simulink model "Backstepping_DELTA"  (R2018b)
settings: Solver=FixedStepAuto  StartTime=0.0  StopTime=25  FixedStep=0.0001  RelTol=1e-5
model workspace (MAT data in the model file):
  I_bc = 0.466666666667
  I_bi = 2.46666666667
  I_brake = 1
  I_m = 1
  R = 0.63
  b = 2
  ee = [0; 0; -2.1944]
  k_r = 1
  l_A = 1
  l_B = 2
  m_b = 1
  m_br = 1.13333333333
  m_c = 0
  m_fb = 0.2
  m_n = 1
  m_nt = 3.6
  m_p = 0
  r_Gb = 0.558823529412
  r_l = 0.63
  r_m = 0.666666666667
  theta = [0 2.09439510239 4.18879020479]
settings Model: Creator=enrico  LastModifiedBy=Dan

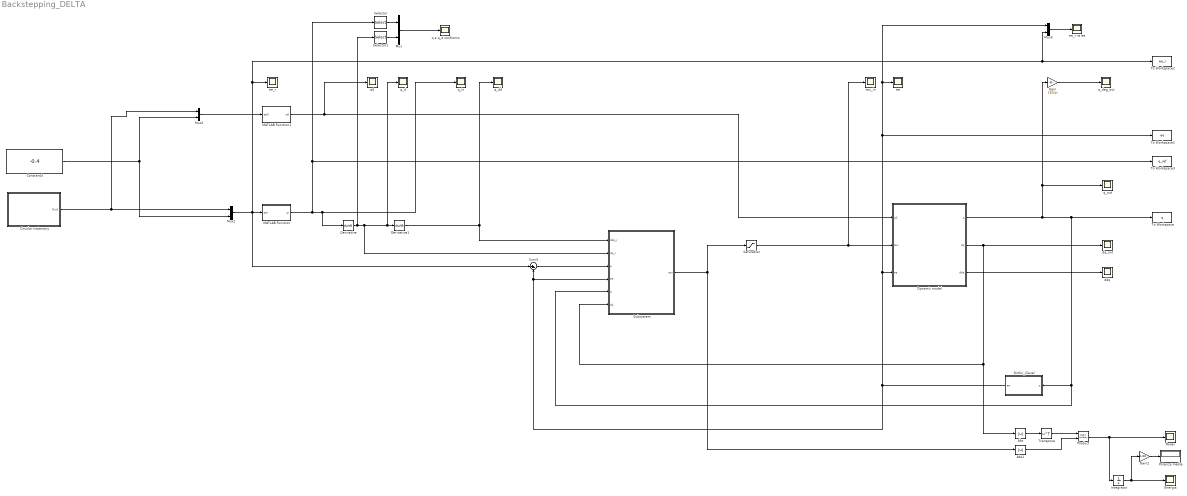
== system Backstepping_DELTA ==
  Abs : Abs
  Abs1 : Abs
  Circular trajectory : Subsystem  mask{A=0.05, F=3}
      mask prompts: A "Amplitude"; F "Frequency"
  Constant3 : Constant  Value=-0.4  SampleTime=-1
  Derivative : Derivative
  Derivative1 : Derivative
  DirKin_Clavel : MATLAB Function  TreatAsAtomicUnit=on
      mask init:
      | loadvar
  Dynamic model : Subsystem
  Energia : Scope
  Gain : Gain  Gain=180/pi
  Gain2 : Gain  Gain=1/10
  Integrator : Integrator
  MATLAB Function : MATLAB Function  TreatAsAtomicUnit=on
  MATLAB Function1 : MATLAB Function  TreatAsAtomicUnit=on
  Mux{,1..3} (4 alike) : Mux  Inputs=2
  Potenza media : Display
  Power : Scope
  Product : Product  Multiplication=Matrix(*)
  Saturation : Saturate  UpperLimit=20  LowerLimit=-20  ZeroCross=off
  Selector : Selector  InputPortWidth=3  IndexOptions=Index vector (dialog)  Indices=[1]  OutputSizes=1
  Selector1 : Selector  InputPortWidth=3  IndexOptions=Index vector (dialog)  Indices=[1]  OutputSizes=1
  Subsystem : Subsystem  mask{K_l=400, K_d=50}
      mask prompts: K_l "Kinematic control gain"; K_d "Derivative_gain"
  Sum3 : Sum  Inputs=|+-
  To Workspace : ToWorkspace  VariableName=q  SampleTime=-1
  To Workspace1 : ToWorkspace  VariableName=ee  SampleTime=-1
  To Workspace2 : ToWorkspace  VariableName=ee_r  SampleTime=-1
  To Workspace3 : ToWorkspace  VariableName=q_ref  SampleTime=-1
  Transpose : Math  Operator=transpose  SaturateOnIntegerOverflow=on
  ddq : Scope
  "dq_out " : Scope
  "ee " : Scope
  ee_r : Scope
  ee_r vs ee : Scope
  q e q_d confronto : Scope
  "q0 " : Scope
  "q_d " : Scope
  q_dd : Scope
  "q_deg_out " : Scope
  q_in : Scope
  q_out : Scope
  tau_in : Scope
  wires:
  Gain/1 -> "q_deg_out "/1
  Dynamic model/3(ddq) -> ddq/1
  Dynamic model/1(q) -> q_out/1, Gain/1, Subsystem/5(q), DirKin_Clavel/1(q), To Workspace/1
  MATLAB Function1/1(q0) -> Dynamic model/1("q0 "), "q0 "/1
  Mux2/1 -> MATLAB Function1/1(ee0)
  Constant3/1 -> Mux1/2, Mux2/2
  Dynamic model/2(dq) -> Abs/1, Subsystem/6(dq), "dq_out "/1
  Subsystem/1(tau) -> Saturation/1, Abs1/1
  Derivative1/1 -> q_dd/1, Subsystem/1(ddq_r)
  Product/1 -> Integrator/1, Power/1
  Transpose/1 -> Product/1
  Abs/1 -> Transpose/1
  Abs1/1 -> Product/2
  Mux/1 -> q e q_d confronto/1
  Selector/1 -> Mux/1
  Selector1/1 -> Mux/2
  MATLAB Function/1(qr) -> Selector/1, To Workspace3/1, q_in/1, Derivative/1
  Derivative/1 -> Derivative1/1, "q_d "/1, Subsystem/2(dq_r), Selector1/1
  DirKin_Clavel/1(ee) -> Mux3/1, "ee "/1, To Workspace1/1, Dynamic model/3(ee), Sum3/2, Subsystem/4(ee)
  Mux3/1 -> ee_r vs ee/1
  Mux1/1 -> MATLAB Function/1(eer), Sum3/1, ee_r/1, To Workspace2/1, Mux3/2
  Integrator/1 -> Gain2/1, Energia/1
  Circular trajectory/1(Out1) -> Mux1/1, Mux2/1
  Gain2/1 -> Potenza media/1
  Sum3/1 -> Subsystem/3(e)
  Saturation/1 -> tau_in/1, Dynamic model/2(tau)

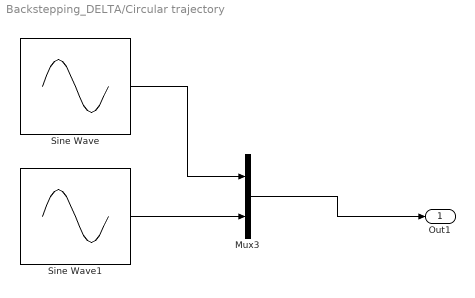
== system Backstepping_DELTA/Circular trajectory ==
  Mux3 : Mux  Inputs=2
  Sine Wave : Sin  Amplitude=A  Frequency=F  Phase=pi/2
  Sine Wave1 : Sin  Amplitude=A  Frequency=F
  Out1 : Outport
  wires:
  Mux3/1 -> Out1/1
  Sine Wave/1 -> Mux3/1
  Sine Wave1/1 -> Mux3/2

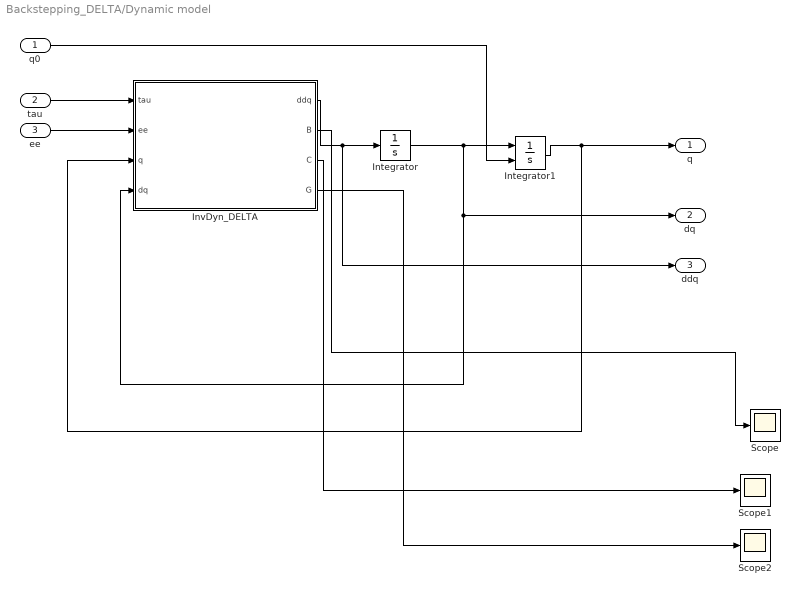
== system Backstepping_DELTA/Dynamic model ==
  "q0 " : Inport
  tau : Inport  Port=2
  ee : Inport  Port=3
  Integrator : Integrator  InitialCondition=[0; 0; 0]
  Integrator1 : Integrator  InitialConditionSource=external  InitialCondition=[pi/4; pi/4; pi/4]
  InvDyn_DELTA : MATLAB Function  TreatAsAtomicUnit=on
  Scope : Scope
  Scope1 : Scope
  Scope2 : Scope
  q : Outport
  dq : Outport  Port=2
  ddq : Outport  Port=3
  wires:
  InvDyn_DELTA/1(ddq) -> ddq/1, Integrator/1
  ee/1 -> InvDyn_DELTA/2(ee)
  Integrator1/1 -> q/1, InvDyn_DELTA/3(q)
  Integrator/1 -> Integrator1/1, dq/1, InvDyn_DELTA/4(dq)
  tau/1 -> InvDyn_DELTA/1(tau)
  "q0 "/1 -> Integrator1/2
  InvDyn_DELTA/2(B) -> Scope/1
  InvDyn_DELTA/3(C) -> Scope1/1
  InvDyn_DELTA/4(G) -> Scope2/1

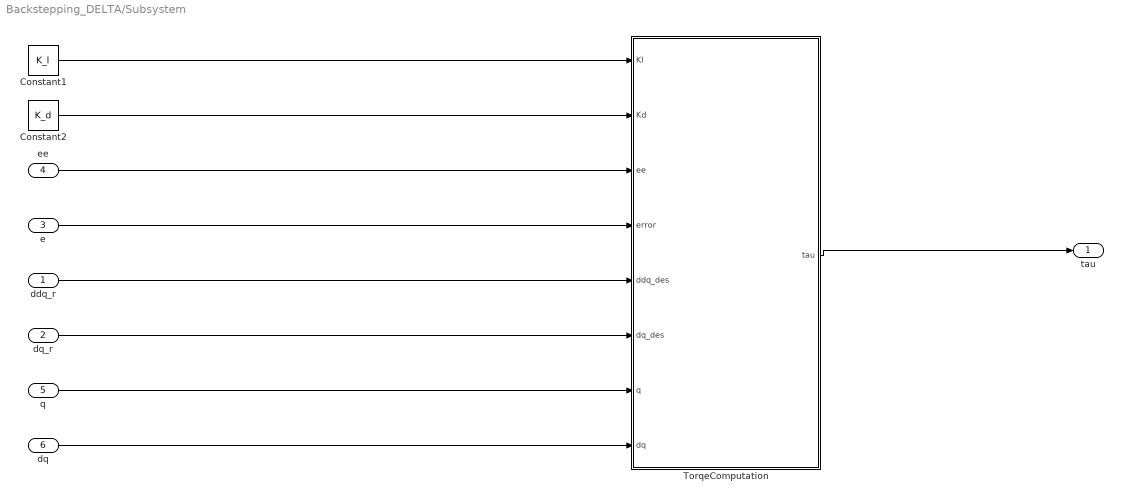
== system Backstepping_DELTA/Subsystem ==
  ddq_r : Inport
  dq_r : Inport  Port=2
  e : Inport  Port=3
  ee : Inport  Port=4
  q : Inport  Port=5
  dq : Inport  Port=6
  Constant1 : Constant  Value=K_l
  Constant2 : Constant  Value=K_d
  TorqeComputation : MATLAB Function  TreatAsAtomicUnit=on
  tau : Outport
  wires:
  ddq_r/1 -> TorqeComputation/5(ddq_des)
  e/1 -> TorqeComputation/4(error)
  q/1 -> TorqeComputation/7(q)
  TorqeComputation/1(tau) -> tau/1
  ee/1 -> TorqeComputation/3(ee)
  dq_r/1 -> TorqeComputation/6(dq_des)
  dq/1 -> TorqeComputation/8(dq)
  Constant1/1 -> TorqeComputation/1(Kl)
  Constant2/1 -> TorqeComputation/2(Kd)

== matlab function Backstepping_DELTA/MATLAB Function1 ==
  data: ee0 input; q0 output
function q0 = InverseKinematic(ee0)
%Computation of the inverse kinematic of the Delta robot

% Loading parameters
[theta, R, ~, ~, l_A, ~, ~, l_B, ~, ~, ~] = Parameters_DELTA;

R_b1 = R_base(theta(1));
R_b2 = R_base(theta(2));
R_b3 = R_base(theta(3));
p = [R_b1\ee0, R_b2\ee0, R_b3\ee0]; 
q0 = nan(3,1);

for li=1:3
    
    x0 = p(1,li);
    y0 = p(2,li);
    z0 = p(3,li);
    A = l_A^2 - l_B^2 - R^2 + x0^2 + y0^2 + z0^2;
    B = 2*x0 - 2*R;

    a = 4*z0^2 + B^2;
    b = 4*R*z0^2 + A*B;
    c = A^2 + 4*R^2*z0^2 - 4*l_A^2*z0^2;
        
    x = (b + sqrt(b^2 - a*c))/a; 
    
    z = (A - B*x)/(2*z0);
    
    q0(li) = - asin(z/l_A); 
    
    if x-R < 0
        q0(li) = pi - q0(li);
    end    
end

end

== matlab function Backstepping_DELTA/Dynamic model/InvDyn_DELTA ==
  data: tau input; ddq output; ee input; q input; dq input; B output; C output; G output
function [ddq, B, C, G] = InvDyn_DELTA(tau, ee, q, dq)
% References:
% [1] Olsson, A. (2009). Modelling and control of a Delta-3 robot, (February).
% [2] Codourey, A. (1998). Dynamic Modeling of Parallel Robots for Computed-Torque Control Implementation, 17(12), 1325–1336.

% B, C, G matrices
[B, C, G, F] = BCG_DELTA(ee,q);


% Inverse dynamic
ddq = B\(tau - C*dq - G - F*dq); % Think adding friction coefficient of the manipulator (from [1] pg 27) 


end

== matlab function Backstepping_DELTA/DirKin_Clavel ==
  data: q input; ee output
function ee = DirKin_Clavel(q)

[theta, R, ~, ~, l_A, ~, ~, l_B, ~, ~, ~] = Parameters_DELTA;

D = nan(3,1);
E = nan(3,1);
F = nan(3,1);
G = nan(3,1);

for i = 1:3
   D(i) = -l_B^2 + l_A^2 + R^2 + 2*R*l_A*cos(q(i));
   
   E(i) = 2*(R + l_A*cos(q(i)))*cos(theta(i));
   
   F(i) = 2*(R + l_A*cos(q(i)))*sin(theta(i));
   
   G(i) = -2*l_A*sin(q(i)); 
end

H = [E(1)*G(2) - E(1)*G(3) - E(2)*G(1) + E(2)*G(3) + E(3)*G(1) - E(3)*G(2);
    -E(1)*F(2) + E(1)*F(3) + E(2)*F(1) - E(2)*F(3) - E(3)*F(1) + E(3)*F(2);
    -E(1)*D(2) + E(1)*D(3) + E(2)*D(1) - E(2)*D(3) - E(3)*D(1) + E(3)*D(2);
     F(1)*D(2) - F(1)*D(3) - F(2)*D(1) + F(2)*D(3) + F(3)*D(1) - F(3)*D(2);
    -F(1)*G(2) + F(1)*G(3) + F(2)*G(1) - F(2)*G(3) - F(3)*G(1) + F(3)*G(2)];

L = (H(5)^2 + H(1)^2)/H(2)^2 + 1;

M = 2*(H(5)*H(4) + H(1)*H(3))/H(2)^2 - (H(5)*E(1) + H(1)*F(1))/H(2) - G(1);

N = (H(4)^2 + H(3)^2)/H(2)^2 - (H(4)*E(1) + H(3)*F(1))/H(2) + D(1);

ee = nan(3,1);
ee2 = nan(3,1);

ee(3) = (-M + sqrt(M^2 - 4*L*N))/(2*L);

ee(1) = ee(3)*H(5)/H(2) + H(4)/H(2);

ee(2) = ee(3)*H(1)/H(2) + H(3)/H(2);

ee2(3) = (-M - sqrt(M^2 - 4*L*N))/(2*L);

ee2(1) = ee2(3)*H(5)/H(2) + H(4)/H(2);

ee2(2) = ee2(3)*H(1)/H(2) + H(3)/H(2);
 


% if ee2(3) < 0 
%     ee = ee2;
% end

if ee(3) > ee2(3)
    ee = ee2;
end

end

== matlab function Backstepping_DELTA/MATLAB Function ==
  data: eer input; qr output
function qr = InverseKinematic(eer)
%Computation of the inverse kinematic of the Delta robot

% Loading parameters
[theta, R, ~, ~, l_A, ~, ~, l_B, ~, ~, ~] = Parameters_DELTA;

R_b1 = R_base(theta(1));
R_b2 = R_base(theta(2));
R_b3 = R_base(theta(3));
p = [R_b1\eer, R_b2\eer, R_b3\eer]; 
qr = nan(3,1);

for li=1:3
    
    x0 = p(1,li);
    y0 = p(2,li);
    z0 = p(3,li);
    A = l_A^2 - l_B^2 - R^2 + x0^2 + y0^2 + z0^2;
    B = 2*x0 - 2*R;

    a = 4*z0^2 + B^2;
    b = 4*R*z0^2 + A*B;
    c = A^2 + 4*R^2*z0^2 - 4*l_A^2*z0^2;
        
    x = (b + sqrt(b^2 - a*c))/a; 
    
    z = (A - B*x)/(2*z0);
    
    qr(li) = - asin(z/l_A); 
    
    if x-R < 0
        qr(li) = pi - qr(li);
    end    
end

end

== matlab function Backstepping_DELTA/Subsystem/TorqeComputation ==
  data: Kl input; Kd input; ee input; error input; ddq_des input; dq_des input; q input; tau output; dq input
% function tau = fcn(ee, e, s, ddq_r, dq_r, q, K_d, K_p)
% 
% [B, C, G, F] = BCG_DELTA(ee,q);
% J = Jacobian_DELTA(ee, q);
% 
% tau = B*ddq_r + F*dq_r + C*dq_r + G + K_d*s + J'*K_p*e;
% 
% end

% For computed torque theory see chapter 2.1.2

function tau  = fcn(Kl, Kd, ee, error, ddq_des, dq_des, q, dq)

% this function compute the B C G matricces of manipulator

Lambda  = Kl*eye(length(q));

d_error = dq - dq_des;

dq_ref  = dq_des - Lambda*error;
ddq_ref = ddq_des - Lambda*d_error;

s = dq - dq_ref;

% Dynamic Matrix function
[B, C, G, F] = BCG_DELTA(ee,q);

[J, ~] = Jacobian_DELTA(ee,q);

% BACKSTEPPING CONTROL (formula 2.29)
tau = B*ddq_ref + C*dq_ref + F*dq_ref + G - Kd*s + J'*error;

end
